simulink model "visitI3A"  (R2023b)
settings: Solver=FixedStepAuto  StartTime=0.0  StopTime=inf  FixedStep=sample_time  RelTol=1e-3
model workspace (MAT data in the model file):
  SL_ROS_VariableLengthArrays_MaxSizes.CommonInfo.ArrayTruncateAction = 'EmitWarning'
  SL_ROS_VariableLengthArrays_MaxSizes.MsgTypeMap = containers.Map
  SL_ROS_VariableLengthArrays_MaxSizes.MsgTypeMap.serialization.keys = {'sensor_msgs/Image'}
  SL_ROS_VariableLengthArrays_MaxSizes.MsgTypeMap.serialization.values{1}(1).PropertyName = 'data'
  SL_ROS_VariableLengthArrays_MaxSizes.MsgTypeMap.serialization.values{1}(1).DataType = 'uint8'
  SL_ROS_VariableLengthArrays_MaxSizes.MsgTypeMap.serialization.values{1}(1).MaxLength = 921600
  SL_ROS_VariableLengthArrays_MaxSizes.MsgTypeMap.serialization.values{1}(2).PropertyName = 'encoding'
  SL_ROS_VariableLengthArrays_MaxSizes.MsgTypeMap.serialization.values{1}(2).DataType = 'uint8'
  SL_ROS_VariableLengthArrays_MaxSizes.MsgTypeMap.serialization.values{1}(2).MaxLength = 128
  SL_ROS_VariableLengthArrays_MaxSizes.MsgTypeMap.serialization.uniformity = 0
  SL_ROS_VariableLengthArrays_MaxSizes.MsgTypeMap.serialization.keyType = 'char'
  SL_ROS_VariableLengthArrays_MaxSizes.MsgTypeMap.serialization.valueType = 'any'
  sample_time = 0.1
undefined symbols (not defined in the file): duration, vel
libraries: ros2lib x16, visionsinks x4, vrlib x4, simulink_extras x4
settings Model: Creator=rcasado  LastModifiedBy=usuario
settings SolverCC: AlgebraicLoopSolver=TrustRegion
settings DataIOCC: ReturnWorkspaceOutputs=off
settings OptimizationCC: EnhancedBackFolding=on  PassReuseOutputArgsAs=Individual arguments  ZeroExternalMemoryAtStartup=off  ZeroInternalMemoryAtStartup=off  MaxStackSize=64  OptimizeBlockOrder=speed  DifferentSizesBufferReuse=on  OptimizationCustomize=off  EfficientTunableParamExpr=on
settings DebuggingCC: ParameterTunabilityLossMsg=error  UnconnectedInputMsg=warning  UnconnectedOutputMsg=warning  UnconnectedLineMsg=warning  BusObjectLabelMismatch=none  PregeneratedLibrarySubsystemCodeDiagnostic=none  ArithmeticOperatorsInVariantConditions=warning
settings HardwareCC: ProdBitPerPointer=32  ProdBitPerSizeT=32  ProdBitPerPtrDiffT=32  ProdLargestAtomicFloat=None  ProdIntDivRoundTo=Undefined  ProdEndianess=Unspecified  ProdWordSize=32  ProdHWDeviceType=Generic->Unspecified (assume 32-bit Generic)
settings ModelReferenceCC: EnableRefExpFcnMdlSchedulingChecks=on
settings SFSimCC: SimUseLocalCustomCode=off  CustomCodeUndefinedFunction=UseInterfaceOnly  SimTargetLang=C++
settings RTWCC: Description=Embedded Coder  SystemTargetFile=ert.tlc  HardwareBoard=Robot Operating System (ROS)  TLCOptions="-aInlineSetEventsForThisBaseRateFcn=TLC_FALSE -aSuppressMultiTaskScheduler=TLC_FALSE  -aRateBasedStepFcn=0"  TemplateMakefile=ert_default_tmf  GenerateReport=on  RTWUseLocalCustomCode=off  Toolchain=Catkin  IncludeHyperlinkInReport=on  LaunchReport=on  TargetLang=C++  GenerateTraceInfo=on  GenerateTraceReport=on  GenerateTraceReportSl=on  GenerateTraceReportSf=on  GenerateTraceReportEml=on  DLArmComputeVersion=19.05
settings CodeAppCC: ForceParamTrailComments=on  IgnoreCustomStorageClasses=off  OperatorAnnotations=on  SimulinkDataObjDesc=on  SFDataObjDesc=on  InsertBlockDesc=on

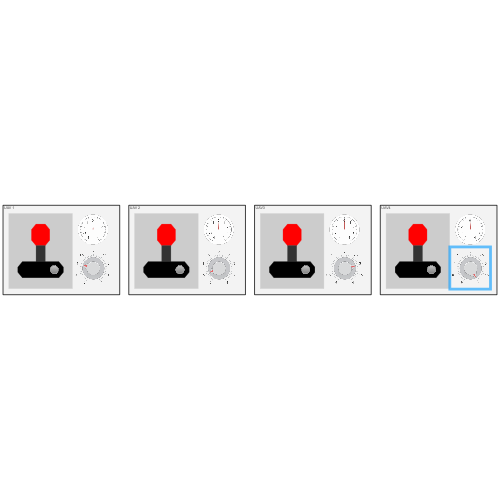
[thumbnail: Simulink's stored preview of the top-level diagram]
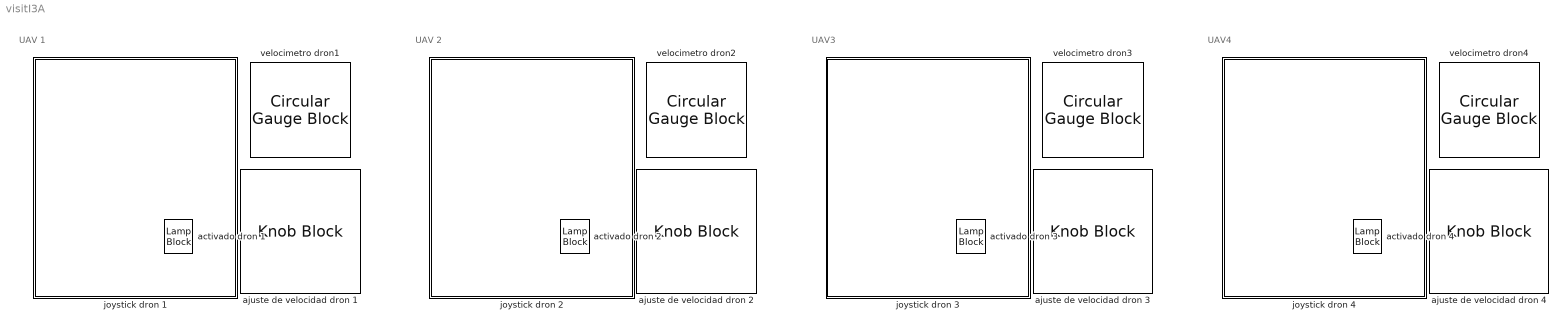
== system visitI3A ==
  note: UAV 1
  note: UAV 2
  note: UAV3
  note: UAV4
  activado dron {1..4} (4 alike) : LampBlock  LabelPosition=Hide
  ajuste de velocidad dron {1..4} (4 alike) : KnobBlock  LabelPosition=Hide  ScaleMax=4  TickInterval=0.5
  joystick dron 1 : Subsystem
      mask Display:
      | patch([12 -2 -2 12], [12 12 -2 -2], [0.8 0.8 0.8])
      | 
      | % bola roja
      | patch([4 6 7 7 6 4 3 3], [6 6 7 9 10 10 9 7], [1 0 0])
      | 
      | % palo gris
      | patch([4 6 6 4], [3 3 6 6], [0.2 0.2 0.2])
      | 
      | % base negra
      | patch([1 9 10 10 9 1 0 0], [0 0 1 2 3 3 2 1], [0 0 0])
  joystick dron 2 : Subsystem
      mask Display:
      | patch([12 -2 -2 12], [12 12 -2 -2], [0.8 0.8 0.8])
      | 
      | % bola roja
      | patch([4 6 7 7 6 4 3 3], [6 6 7 9 10 10 9 7], [1 0 0])
      | 
      | % palo gris
      | patch([4 6 6 4], [3 3 6 6], [0.2 0.2 0.2])
      | 
      | % base negra
      | patch([1 9 10 10 9 1 0 0], [0 0 1 2 3 3 2 1], [0 0 0])
  joystick dron 3 : Subsystem
      mask Display:
      | patch([12 -2 -2 12], [12 12 -2 -2], [0.8 0.8 0.8])
      | 
      | % bola roja
      | patch([4 6 7 7 6 4 3 3], [6 6 7 9 10 10 9 7], [1 0 0])
      | 
      | % palo gris
      | patch([4 6 6 4], [3 3 6 6], [0.2 0.2 0.2])
      | 
      | % base negra
      | patch([1 9 10 10 9 1 0 0], [0 0 1 2 3 3 2 1], [0 0 0])
  joystick dron 4 : Subsystem
      mask Display:
      | patch([12 -2 -2 12], [12 12 -2 -2], [0.8 0.8 0.8])
      | 
      | % bola roja
      | patch([4 6 7 7 6 4 3 3], [6 6 7 9 10 10 9 7], [1 0 0])
      | 
      | % palo gris
      | patch([4 6 6 4], [3 3 6 6], [0.2 0.2 0.2])
      | 
      | % base negra
      | patch([1 9 10 10 9 1 0 0], [0 0 1 2 3 3 2 1], [0 0 0])
  velocimetro dron{1..4} (4 alike) : CircularGaugeBlock  LabelPosition=Hide  ScaleMin=-4  ScaleMax=4  TickInterval=1

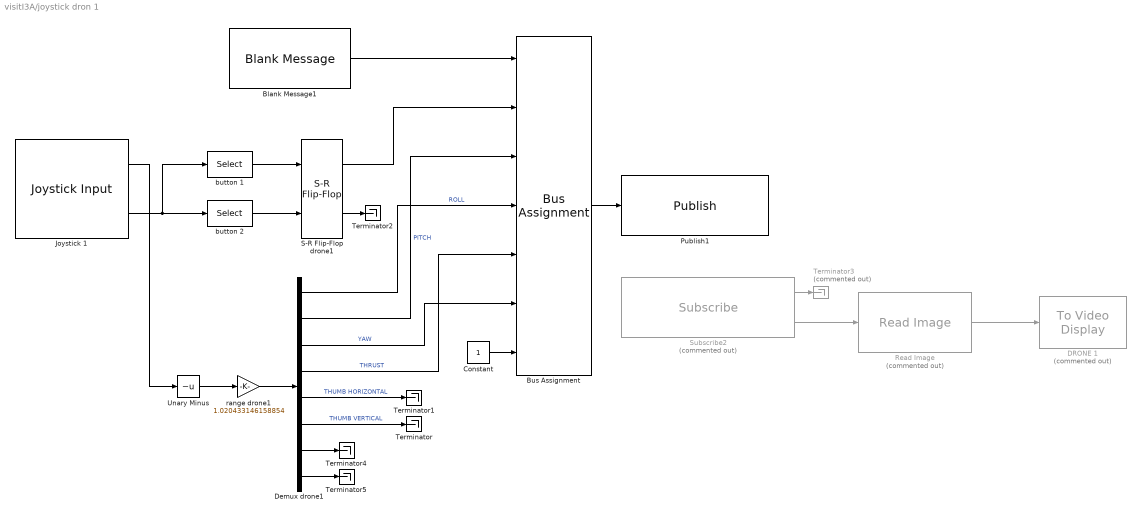
== system visitI3A/joystick dron 1 ==
  Blank Message1 : ros2lib/Blank Message  messageClass=Message  entityType=navsim_msgs/RemoteCommand  messageType=navsim_msgs/RemoteCommand  SampleTime=sample_time
  Bus Assignment : BusAssignment  AssignedSignals=on,vel.linear.x,vel.linear.y,vel.linear.z,vel.angular.z,duration.sec
  Constant : Constant  OutDataTypeStr=int32
  DRONE 1 : visionsinks/To Video Display  Commented=on  windowSizeMode=True size (1:1)  openAtMdlStart=on  fullScreen=off  videoWindowX=536805376  videoWindowY=536805376  saveWindowSize=off  videoWindowWidth=480  videoWindowHeight=320  inputColorFormat=RGB  inputType=Obsolete  imagePorts=One multidimensional signal  OutputDevice=On-screen video monitor  dataOrg=Column-major  isWindowOpen=off
  Demux drone1 : Demux  Outputs=8
  Joystick 1 : vrlib/Joystick Input  joyid=2  adjustports=off  forcefeed=off
  Publish1 : ros2lib/Publish  topicSource=Select from ROS network  topic=/NavSim/abejorro1/RemoteCommand  messageType=navsim_msgs/RemoteCommand  QOSHistory=Keep last  QOSDepth=1  QOSReliability=Reliable  QOSDurability=Volatile
  Read Image : ros2lib/Read Image  Commented=on  MaximumImageSize=[320, 480]  ImageEncoding=rgb8  ShowAlphaOutput=off  ShowErrorCodeOutput=off  VariableSizeOutputs=off
  S-R Flip-Flop drone1 : simulink_extras/Flip Flops/S-R Flip-Flop  initial_condition=0
  Subscribe2 : ros2lib/Subscribe  Commented=on  topicSource=Select from ROS network  topic=/NavSim/abejorro1/follow_cam/image_raw  messageType=sensor_msgs/Image  sampleTime=0.1  QOSHistory=Keep last  QOSDepth=1  QOSReliability=Reliable  QOSDurability=Volatile
  Terminator{,1..2,4..5} (5 alike) : Terminator
  Terminator3 : Terminator  Commented=on
  Unary Minus : UnaryMinus
  button 1 : Selector  InputPortWidth=32  IndexOptions=Index vector (dialog)  Indices=[1]  OutputSizes=1
  button 2 : Selector  InputPortWidth=32  IndexOptions=Index vector (dialog)  Indices=[2]  OutputSizes=1
  range drone1 : Gain  Gain=1.020433146158854
  wires:
  Bus Assignment/1 -> Publish1/1
  Blank Message1/1 -> Bus Assignment/1
  Joystick 1/1 -> Unary Minus/1
  Demux drone1/1 -> Bus Assignment/4  "ROLL"
  Demux drone1/2 -> Bus Assignment/3  "PITCH"
  Demux drone1/3 -> Bus Assignment/6  "YAW"
  Demux drone1/4 -> Bus Assignment/5  "THRUST"
  Demux drone1/5 -> Terminator1/1  "THUMB HORIZONTAL"
  Demux drone1/6 -> Terminator/1  "THUMB VERTICAL"
  Demux drone1/7 -> Terminator4/1
  Demux drone1/8 -> Terminator5/1
  Joystick 1/2 -> button 2/1, button 1/1
  S-R Flip-Flop drone1/1 -> Bus Assignment/2
  button 2/1 -> S-R Flip-Flop drone1/2
  button 1/1 -> S-R Flip-Flop drone1/1
  S-R Flip-Flop drone1/2 -> Terminator2/1
  Unary Minus/1 -> range drone1/1
  range drone1/1 -> Demux drone1/1
  Subscribe2/1 -> Terminator3/1
  Subscribe2/2 -> Read Image/1
  Read Image/1 -> DRONE 1/1
  Constant/1 -> Bus Assignment/7

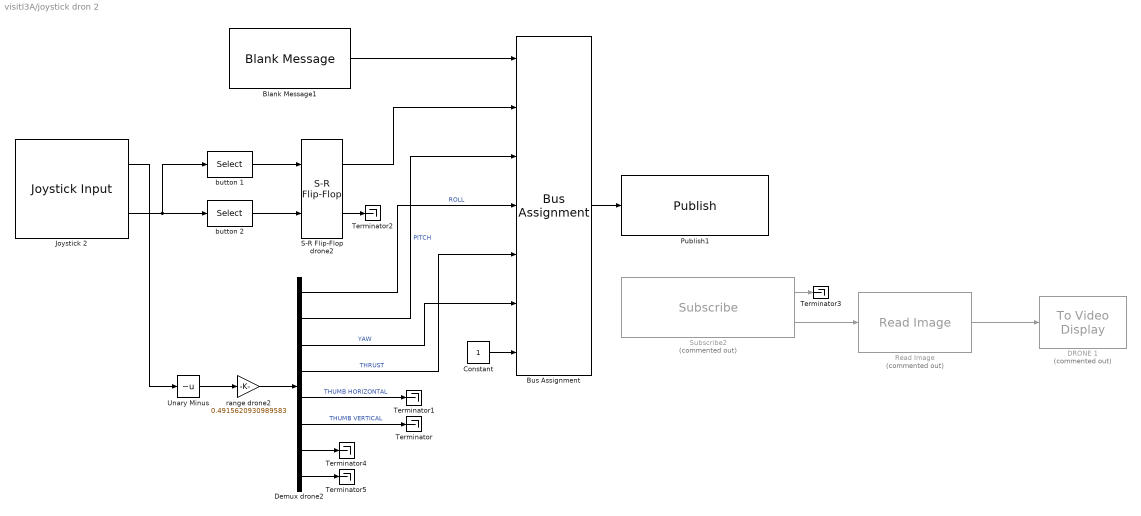
== system visitI3A/joystick dron 2 ==
  Blank Message1 : ros2lib/Blank Message  messageClass=Message  entityType=navsim_msgs/RemoteCommand  messageType=navsim_msgs/RemoteCommand  SampleTime=sample_time
  Bus Assignment : BusAssignment  AssignedSignals=on,vel.linear.x,vel.linear.y,vel.linear.z,vel.angular.z,duration.sec
  Constant : Constant  OutDataTypeStr=int32
  DRONE 1 : visionsinks/To Video Display  Commented=on  windowSizeMode=True size (1:1)  openAtMdlStart=on  fullScreen=off  videoWindowX=536805376  videoWindowY=536805376  saveWindowSize=off  videoWindowWidth=480  videoWindowHeight=320  inputColorFormat=RGB  inputType=Obsolete  imagePorts=One multidimensional signal  OutputDevice=On-screen video monitor  dataOrg=Column-major  isWindowOpen=off
  Demux drone2 : Demux  Outputs=8
  Joystick 2 : vrlib/Joystick Input  joyid=3  adjustports=off  forcefeed=off
  Publish1 : ros2lib/Publish  topicSource=Select from ROS network  topic=/NavSim/abejorro2/RemoteCommand  messageType=navsim_msgs/RemoteCommand  QOSHistory=Keep last  QOSDepth=1  QOSReliability=Reliable  QOSDurability=Volatile
  Read Image : ros2lib/Read Image  Commented=on  MaximumImageSize=[320, 480]  ImageEncoding=rgb8  ShowAlphaOutput=off  ShowErrorCodeOutput=off  VariableSizeOutputs=off
  S-R Flip-Flop drone2 : simulink_extras/Flip Flops/S-R Flip-Flop  initial_condition=0
  Subscribe2 : ros2lib/Subscribe  Commented=on  topicSource=Select from ROS network  topic=/NavSim/abejorro2/follow_cam/image_raw  messageType=sensor_msgs/Image  sampleTime=0.1  QOSHistory=Keep last  QOSDepth=1  QOSReliability=Reliable  QOSDurability=Volatile
  Terminator{,1..5} (6 alike) : Terminator
  Unary Minus : UnaryMinus
  button 1 : Selector  InputPortWidth=32  IndexOptions=Index vector (dialog)  Indices=[1]  OutputSizes=1
  button 2 : Selector  InputPortWidth=32  IndexOptions=Index vector (dialog)  Indices=[2]  OutputSizes=1
  range drone2 : Gain  Gain=0.4915620930989583
  wires:
  Bus Assignment/1 -> Publish1/1
  Blank Message1/1 -> Bus Assignment/1
  Joystick 2/1 -> Unary Minus/1
  Demux drone2/1 -> Bus Assignment/4  "ROLL"
  Demux drone2/2 -> Bus Assignment/3  "PITCH"
  Demux drone2/3 -> Bus Assignment/6  "YAW"
  Demux drone2/4 -> Bus Assignment/5  "THRUST"
  Demux drone2/5 -> Terminator1/1  "THUMB HORIZONTAL"
  Demux drone2/6 -> Terminator/1  "THUMB VERTICAL"
  Demux drone2/7 -> Terminator4/1
  Demux drone2/8 -> Terminator5/1
  Joystick 2/2 -> button 2/1, button 1/1
  S-R Flip-Flop drone2/1 -> Bus Assignment/2
  button 2/1 -> S-R Flip-Flop drone2/2
  button 1/1 -> S-R Flip-Flop drone2/1
  S-R Flip-Flop drone2/2 -> Terminator2/1
  Unary Minus/1 -> range drone2/1
  range drone2/1 -> Demux drone2/1
  Subscribe2/1 -> Terminator3/1
  Subscribe2/2 -> Read Image/1
  Read Image/1 -> DRONE 1/1
  Constant/1 -> Bus Assignment/7

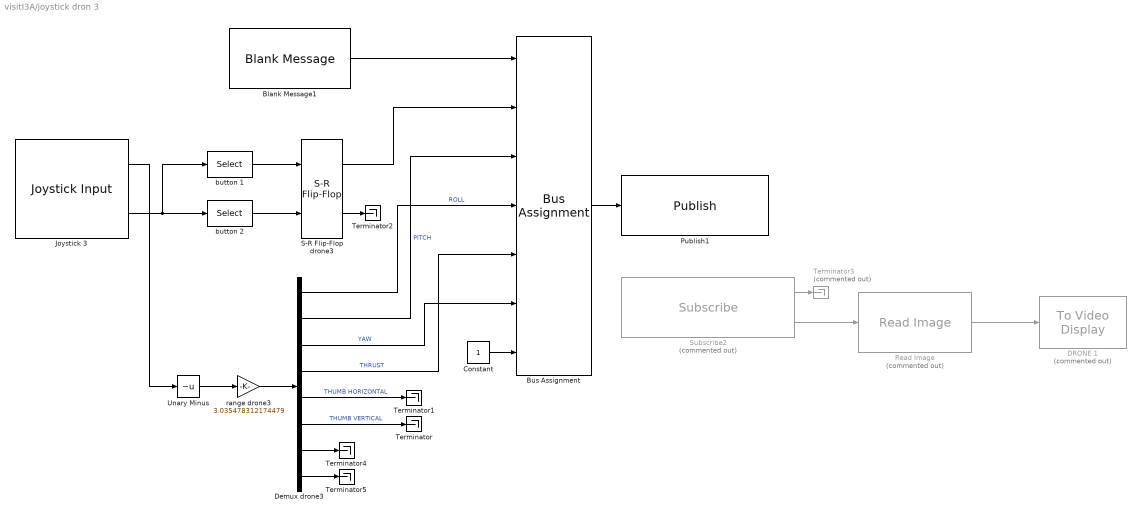
== system visitI3A/joystick dron 3 ==
  Blank Message1 : ros2lib/Blank Message  messageClass=Message  entityType=navsim_msgs/RemoteCommand  messageType=navsim_msgs/RemoteCommand  SampleTime=sample_time
  Bus Assignment : BusAssignment  AssignedSignals=on,vel.linear.x,vel.linear.y,vel.linear.z,vel.angular.z,duration.sec
  Constant : Constant  OutDataTypeStr=int32
  DRONE 1 : visionsinks/To Video Display  Commented=on  windowSizeMode=True size (1:1)  openAtMdlStart=on  fullScreen=off  videoWindowX=536805376  videoWindowY=536805376  saveWindowSize=off  videoWindowWidth=480  videoWindowHeight=320  inputColorFormat=RGB  inputType=Obsolete  imagePorts=One multidimensional signal  OutputDevice=On-screen video monitor  dataOrg=Column-major  isWindowOpen=off
  Demux drone3 : Demux  Outputs=8
  Joystick 3 : vrlib/Joystick Input  joyid=4  adjustports=off  forcefeed=off
  Publish1 : ros2lib/Publish  topicSource=Select from ROS network  topic=/NavSim/abejorro3/RemoteCommand  messageType=navsim_msgs/RemoteCommand  QOSHistory=Keep last  QOSDepth=1  QOSReliability=Reliable  QOSDurability=Volatile
  Read Image : ros2lib/Read Image  Commented=on  MaximumImageSize=[320, 480]  ImageEncoding=rgb8  ShowAlphaOutput=off  ShowErrorCodeOutput=off  VariableSizeOutputs=off
  S-R Flip-Flop drone3 : simulink_extras/Flip Flops/S-R Flip-Flop  initial_condition=0
  Subscribe2 : ros2lib/Subscribe  Commented=on  topicSource=Select from ROS network  topic=/NavSim/abejorro3/follow_cam/image_raw  messageType=sensor_msgs/Image  sampleTime=0.1  QOSHistory=Keep last  QOSDepth=1  QOSReliability=Reliable  QOSDurability=Volatile
  Terminator{,1..2,4..5} (5 alike) : Terminator
  Terminator3 : Terminator  Commented=on
  Unary Minus : UnaryMinus
  button 1 : Selector  InputPortWidth=32  IndexOptions=Index vector (dialog)  Indices=[1]  OutputSizes=1
  button 2 : Selector  InputPortWidth=32  IndexOptions=Index vector (dialog)  Indices=[2]  OutputSizes=1
  range drone3 : Gain  Gain=3.035478312174479
  wires:
  Bus Assignment/1 -> Publish1/1
  Blank Message1/1 -> Bus Assignment/1
  Joystick 3/1 -> Unary Minus/1
  Demux drone3/1 -> Bus Assignment/4  "ROLL"
  Demux drone3/2 -> Bus Assignment/3  "PITCH"
  Demux drone3/3 -> Bus Assignment/6  "YAW"
  Demux drone3/4 -> Bus Assignment/5  "THRUST"
  Demux drone3/5 -> Terminator1/1  "THUMB HORIZONTAL"
  Demux drone3/6 -> Terminator/1  "THUMB VERTICAL"
  Demux drone3/7 -> Terminator4/1
  Demux drone3/8 -> Terminator5/1
  Joystick 3/2 -> button 2/1, button 1/1
  S-R Flip-Flop drone3/1 -> Bus Assignment/2
  button 2/1 -> S-R Flip-Flop drone3/2
  button 1/1 -> S-R Flip-Flop drone3/1
  S-R Flip-Flop drone3/2 -> Terminator2/1
  Unary Minus/1 -> range drone3/1
  range drone3/1 -> Demux drone3/1
  Subscribe2/1 -> Terminator3/1
  Subscribe2/2 -> Read Image/1
  Read Image/1 -> DRONE 1/1
  Constant/1 -> Bus Assignment/7

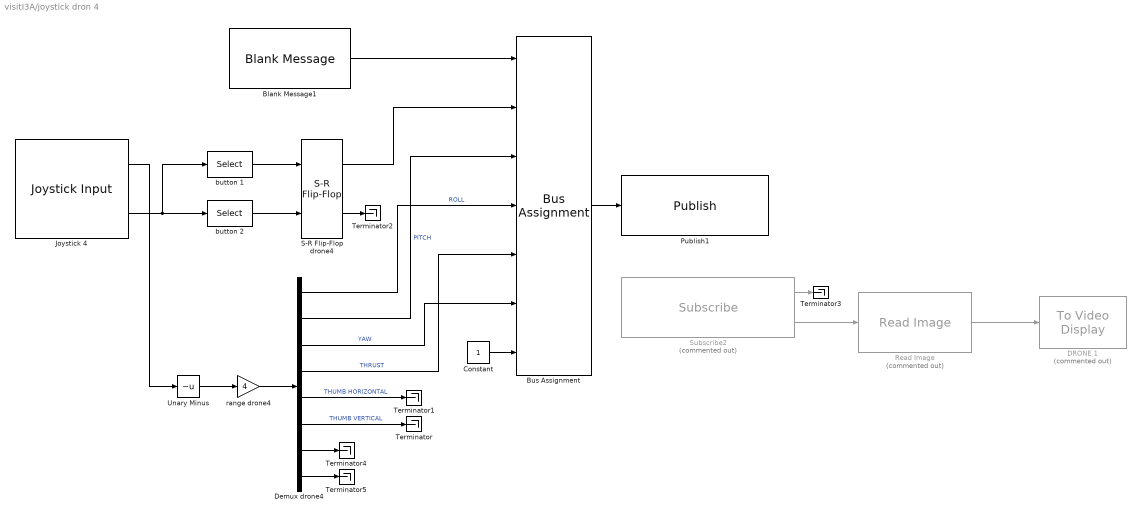
== system visitI3A/joystick dron 4 ==
  Blank Message1 : ros2lib/Blank Message  messageClass=Message  entityType=navsim_msgs/RemoteCommand  messageType=navsim_msgs/RemoteCommand  SampleTime=sample_time
  Bus Assignment : BusAssignment  AssignedSignals=on,vel.linear.x,vel.linear.y,vel.linear.z,vel.angular.z,duration.sec
  Constant : Constant  OutDataTypeStr=int32
  DRONE 1 : visionsinks/To Video Display  Commented=on  windowSizeMode=True size (1:1)  openAtMdlStart=on  fullScreen=off  videoWindowX=536805376  videoWindowY=536805376  saveWindowSize=off  videoWindowWidth=480  videoWindowHeight=320  inputColorFormat=RGB  inputType=Obsolete  imagePorts=One multidimensional signal  OutputDevice=On-screen video monitor  dataOrg=Column-major  isWindowOpen=off
  Demux drone4 : Demux  Outputs=8
  Joystick 4 : vrlib/Joystick Input  joyid=1  adjustports=off  forcefeed=off
  Publish1 : ros2lib/Publish  topicSource=Select from ROS network  topic=/NavSim/abejorro4/RemoteCommand  messageType=navsim_msgs/RemoteCommand  QOSHistory=Keep last  QOSDepth=1  QOSReliability=Reliable  QOSDurability=Volatile
  Read Image : ros2lib/Read Image  Commented=on  MaximumImageSize=[320, 480]  ImageEncoding=rgb8  ShowAlphaOutput=off  ShowErrorCodeOutput=off  VariableSizeOutputs=off
  S-R Flip-Flop drone4 : simulink_extras/Flip Flops/S-R Flip-Flop  initial_condition=0
  Subscribe2 : ros2lib/Subscribe  Commented=on  topicSource=Select from ROS network  topic=/NavSim/abejorro4/follow_cam/image_raw  messageType=sensor_msgs/Image  sampleTime=0.1  QOSHistory=Keep last  QOSDepth=1  QOSReliability=Reliable  QOSDurability=Volatile
  Terminator{,1..5} (6 alike) : Terminator
  Unary Minus : UnaryMinus
  button 1 : Selector  InputPortWidth=32  IndexOptions=Index vector (dialog)  Indices=[1]  OutputSizes=1
  button 2 : Selector  InputPortWidth=32  IndexOptions=Index vector (dialog)  Indices=[2]  OutputSizes=1
  range drone4 : Gain  Gain=4
  wires:
  Bus Assignment/1 -> Publish1/1
  Blank Message1/1 -> Bus Assignment/1
  Joystick 4/1 -> Unary Minus/1
  Demux drone4/1 -> Bus Assignment/4  "ROLL"
  Demux drone4/2 -> Bus Assignment/3  "PITCH"
  Demux drone4/3 -> Bus Assignment/6  "YAW"
  Demux drone4/4 -> Bus Assignment/5  "THRUST"
  Demux drone4/5 -> Terminator1/1  "THUMB HORIZONTAL"
  Demux drone4/6 -> Terminator/1  "THUMB VERTICAL"
  Demux drone4/7 -> Terminator4/1
  Demux drone4/8 -> Terminator5/1
  Joystick 4/2 -> button 2/1, button 1/1
  S-R Flip-Flop drone4/1 -> Bus Assignment/2
  button 2/1 -> S-R Flip-Flop drone4/2
  button 1/1 -> S-R Flip-Flop drone4/1
  S-R Flip-Flop drone4/2 -> Terminator2/1
  Unary Minus/1 -> range drone4/1
  range drone4/1 -> Demux drone4/1
  Subscribe2/1 -> Terminator3/1
  Subscribe2/2 -> Read Image/1
  Read Image/1 -> DRONE 1/1
  Constant/1 -> Bus Assignment/7
